simulink model "Add_Frame"  (R2013b)
settings: Solver=FixedStepDiscrete  StartTime=0.0  StopTime=200  RelTol=1e-3
InitFcn:
  | %% DSPBuilder Start
  | alt_dspbuilder_update_model(bdroot)
  | %% DSPBuilder End
StopFcn:
  | ed_out_script
undefined symbols (not defined in the file or in its folder): sigbuilder_block
libraries: allblocks_alteradspbuilder2 x118, simulink x5
(part 2 of 2)

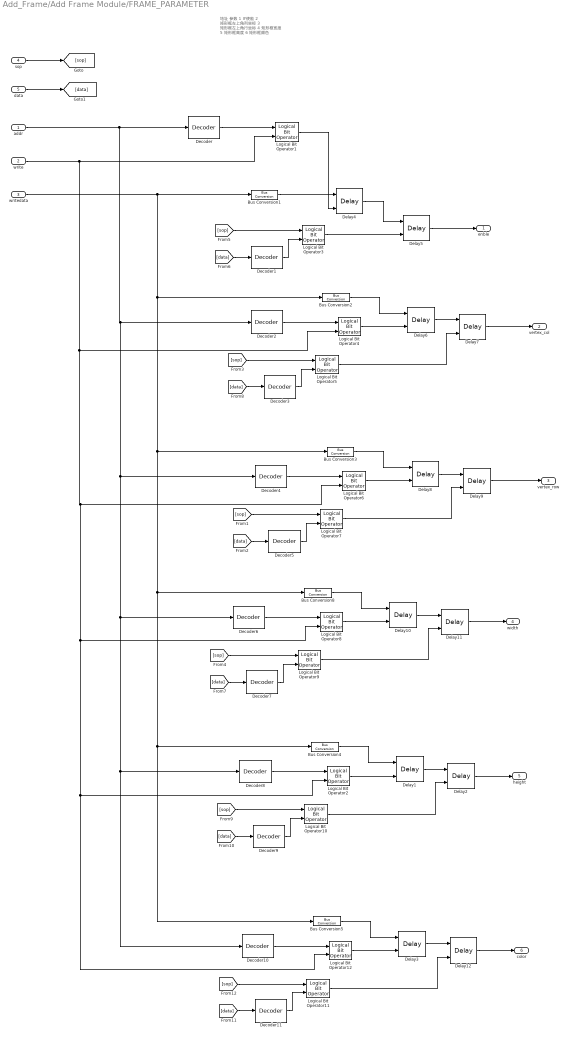
== system Add_Frame/Add Frame Module/FRAME_PARAMETER ==
  note: 地址	参数
      | 1		IP使能
      | 2		矩形框左上角列坐标
      | 3		矩形框左上角行坐标
      | 4		矩形框宽度
      | 5		矩形框高度
      | 6		矩形框颜色
  addr : Inport
  write : Inport  Port=2
  writedata : Inport  Port=3
  sop : Inport  Port=4
  data : Inport  Port=5
  Bus Conversion1 : allblocks_alteradspbuilder2/Bus Conversion  BusType=Unsigned Integer  ibwl=32  ibwr=1  bwl=1  bwr=1  bitToConnectToOutputLSB=0  round=off  saturate=off  pipeline_display=0
  Bus Conversion{2..4,8} (4 alike) : allblocks_alteradspbuilder2/Bus Conversion  BusType=Unsigned Integer  ibwl=32  ibwr=1  bwl=16  bwr=1  bitToConnectToOutputLSB=0  round=off  saturate=off  pipeline_display=0
  Bus Conversion5 : allblocks_alteradspbuilder2/Bus Conversion  BusType=Unsigned Integer  ibwl=32  ibwr=1  bwl=3  bwr=1  bitToConnectToOutputLSB=0  round=off  saturate=off  pipeline_display=0
  Decoder : allblocks_alteradspbuilder2/Decoder  BusType=Unsigned Integer  bwl=3  bwr=2  registered=on  pipeline_display=1  value=1
  Decoder{1,3,5,7,9,11} (6 alike) : allblocks_alteradspbuilder2/Decoder  BusType=Unsigned Integer  bwl=24  bwr=2  registered=off  pipeline_display=0  value=15
  Decoder10 : allblocks_alteradspbuilder2/Decoder  BusType=Unsigned Integer  bwl=3  bwr=2  registered=on  pipeline_display=1  value=6
  Decoder2 : allblocks_alteradspbuilder2/Decoder  BusType=Unsigned Integer  bwl=3  bwr=2  registered=on  pipeline_display=1  value=2
  Decoder4 : allblocks_alteradspbuilder2/Decoder  BusType=Unsigned Integer  bwl=3  bwr=2  registered=on  pipeline_display=1  value=3
  Decoder6 : allblocks_alteradspbuilder2/Decoder  BusType=Unsigned Integer  bwl=3  bwr=2  registered=on  pipeline_display=1  value=4
  Decoder8 : allblocks_alteradspbuilder2/Decoder  BusType=Unsigned Integer  bwl=3  bwr=2  registered=on  pipeline_display=1  value=5
  Delay1 : allblocks_alteradspbuilder2/Delay  pipeline=1  pipeline_display=1  ClockPhase=1  use_ena=on  use_sclr=off  allowFloatingPointOverride=on  logOutputs=off  logFile=E:\FPGA\SOC\Quartus\quartus\dsp_builder\design\VIP_LIB\Add_Frame\tb_Add_Frame\Add%5FFrame_Add+Frame+Module_FRAME%5FPARAMETER_Delay1.fixedpointlog  use_init=on  reset_value=10
  Delay10 : allblocks_alteradspbuilder2/Delay  pipeline=1  pipeline_display=1  ClockPhase=1  use_ena=on  use_sclr=off  allowFloatingPointOverride=on  logOutputs=off  logFile=E:\FPGA\SOC\Quartus\quartus\dsp_builder\design\VIP_LIB\Add_Frame\tb_Add_Frame\Add%5FFrame_Add+Frame+Module_FRAME%5FPARAMETER_Delay10.fixedpointlog  use_init=on  reset_value=10
  Delay11 : allblocks_alteradspbuilder2/Delay  pipeline=1  pipeline_display=1  ClockPhase=1  use_ena=on  use_sclr=off  allowFloatingPointOverride=on  logOutputs=off  logFile=E:\FPGA\SOC\Quartus\quartus\dsp_builder\design\VIP_LIB\Add_Frame\tb_Add_Frame\Add%5FFrame_Add+Frame+Module_FRAME%5FPARAMETER_Delay11.fixedpointlog  use_init=on  reset_value=10
  Delay12 : allblocks_alteradspbuilder2/Delay  pipeline=1  pipeline_display=1  ClockPhase=1  use_ena=on  use_sclr=off  allowFloatingPointOverride=on  logOutputs=off  logFile=E:\FPGA\SOC\Quartus\quartus\dsp_builder\design\VIP_LIB\Add_Frame\tb_Add_Frame\Add%5FFrame_Add+Frame+Module_FRAME%5FPARAMETER_Delay12.fixedpointlog  use_init=on  reset_value=0
  Delay2 : allblocks_alteradspbuilder2/Delay  pipeline=1  pipeline_display=1  ClockPhase=1  use_ena=on  use_sclr=off  allowFloatingPointOverride=on  logOutputs=off  logFile=E:\FPGA\SOC\Quartus\quartus\dsp_builder\design\VIP_LIB\Add_Frame\tb_Add_Frame\Add%5FFrame_Add+Frame+Module_FRAME%5FPARAMETER_Delay2.fixedpointlog  use_init=on  reset_value=10
  Delay3 : allblocks_alteradspbuilder2/Delay  pipeline=1  pipeline_display=1  ClockPhase=1  use_ena=on  use_sclr=off  allowFloatingPointOverride=on  logOutputs=off  logFile=E:\FPGA\SOC\Quartus\quartus\dsp_builder\design\VIP_LIB\Add_Frame\tb_Add_Frame\Add%5FFrame_Add+Frame+Module_FRAME%5FPARAMETER_Delay3.fixedpointlog  use_init=on  reset_value=0
  Delay4 : allblocks_alteradspbuilder2/Delay  pipeline=1  pipeline_display=1  ClockPhase=1  use_ena=on  use_sclr=off  allowFloatingPointOverride=on  logOutputs=off  logFile=E:\FPGA\SOC\Quartus\quartus\dsp_builder\design\VIP_LIB\Add_Frame\tb_Add_Frame\Add%5FFrame_Add+Frame+Module_FRAME%5FPARAMETER_Delay4.fixedpointlog  use_init=on  reset_value=0
  Delay5 : allblocks_alteradspbuilder2/Delay  pipeline=1  pipeline_display=1  ClockPhase=1  use_ena=on  use_sclr=off  allowFloatingPointOverride=on  logOutputs=off  logFile=E:\FPGA\SOC\Quartus\quartus\dsp_builder\design\VIP_LIB\Add_Frame\tb_Add_Frame\Add%5FFrame_Add+Frame+Module_FRAME%5FPARAMETER_Delay5.fixedpointlog  use_init=on  reset_value=0
  Delay6 : allblocks_alteradspbuilder2/Delay  pipeline=1  pipeline_display=1  ClockPhase=1  use_ena=on  use_sclr=off  allowFloatingPointOverride=on  logOutputs=off  logFile=E:\FPGA\SOC\Quartus\quartus\dsp_builder\design\VIP_LIB\Add_Frame\tb_Add_Frame\Add%5FFrame_Add+Frame+Module_FRAME%5FPARAMETER_Delay6.fixedpointlog  use_init=on  reset_value=10
  Delay7 : allblocks_alteradspbuilder2/Delay  pipeline=1  pipeline_display=1  ClockPhase=1  use_ena=on  use_sclr=off  allowFloatingPointOverride=on  logOutputs=off  logFile=E:\FPGA\SOC\Quartus\quartus\dsp_builder\design\VIP_LIB\Add_Frame\tb_Add_Frame\Add%5FFrame_Add+Frame+Module_FRAME%5FPARAMETER_Delay7.fixedpointlog  use_init=on  reset_value=10
  Delay8 : allblocks_alteradspbuilder2/Delay  pipeline=1  pipeline_display=1  ClockPhase=1  use_ena=on  use_sclr=off  allowFloatingPointOverride=on  logOutputs=off  logFile=E:\FPGA\SOC\Quartus\quartus\dsp_builder\design\VIP_LIB\Add_Frame\tb_Add_Frame\Add%5FFrame_Add+Frame+Module_FRAME%5FPARAMETER_Delay8.fixedpointlog  use_init=on  reset_value=10
  Delay9 : allblocks_alteradspbuilder2/Delay  pipeline=1  pipeline_display=1  ClockPhase=1  use_ena=on  use_sclr=off  allowFloatingPointOverride=on  logOutputs=off  logFile=E:\FPGA\SOC\Quartus\quartus\dsp_builder\design\VIP_LIB\Add_Frame\tb_Add_Frame\Add%5FFrame_Add+Frame+Module_FRAME%5FPARAMETER_Delay9.fixedpointlog  use_init=on  reset_value=10
  Logical Bit Operator{1..12} (12 alike) : allblocks_alteradspbuilder2/Logical Bit Operator  LogicalOperator=AND  user_inputs=2  pipeline_display=0
  enble : Outport
  vertex_col : Outport  Port=2
  vertex_row : Outport  Port=3
  width : Outport  Port=4
  height : Outport  Port=5
  color : Outport  Port=6
  wires:
  Decoder/1 -> Logical Bit Operator1/1
  [data] -> Decoder1/1
  [sop] -> Logical Bit Operator3/1
  Decoder1/1 -> Logical Bit Operator3/2
  Logical Bit Operator1/1 -> Delay4/2
  Logical Bit Operator3/1 -> Delay5/2
  Bus Conversion1/1 -> Delay4/1
  Decoder2/1 -> Logical Bit Operator4/1
  Delay6/1 -> Delay7/1
  [data] -> Decoder3/1
  [sop] -> Logical Bit Operator5/1
  Decoder3/1 -> Logical Bit Operator5/2
  Logical Bit Operator4/1 -> Delay6/2
  Bus Conversion2/1 -> Delay6/1
  Decoder4/1 -> Logical Bit Operator6/1
  [data] -> Decoder5/1
  [sop] -> Logical Bit Operator7/1
  Decoder5/1 -> Logical Bit Operator7/2
  Logical Bit Operator7/1 -> Delay9/2
  Logical Bit Operator6/1 -> Delay8/2
  Bus Conversion3/1 -> Delay8/1
  writedata/1 -> Bus Conversion5/1, Bus Conversion4/1, Bus Conversion8/1, Bus Conversion3/1, Bus Conversion2/1, Bus Conversion1/1
  Decoder6/1 -> Logical Bit Operator8/1
  Delay10/1 -> Delay11/1
  [data] -> Decoder7/1
  [sop] -> Logical Bit Operator9/1
  Decoder7/1 -> Logical Bit Operator9/2
  Logical Bit Operator9/1 -> Delay11/2
  Logical Bit Operator8/1 -> Delay10/2
  Bus Conversion8/1 -> Delay10/1
  sop/1 -> [sop]
  data/1 -> [data]
  Delay4/1 -> Delay5/1
  Delay5/1 -> enble/1
  Logical Bit Operator5/1 -> Delay7/2
  Delay7/1 -> vertex_col/1
  Delay8/1 -> Delay9/1
  Delay9/1 -> vertex_row/1
  Delay11/1 -> width/1
  Decoder8/1 -> Logical Bit Operator2/1
  Delay1/1 -> Delay2/1
  [data] -> Decoder9/1
  [sop] -> Logical Bit Operator10/1
  Decoder9/1 -> Logical Bit Operator10/2
  Logical Bit Operator10/1 -> Delay2/2
  Logical Bit Operator2/1 -> Delay1/2
  Bus Conversion4/1 -> Delay1/1
  Delay2/1 -> height/1
  write/1 -> Logical Bit Operator1/2, Logical Bit Operator12/2, Logical Bit Operator2/2, Logical Bit Operator8/2, Logical Bit Operator6/2, Logical Bit Operator4/2
  Decoder10/1 -> Logical Bit Operator12/1
  Delay3/1 -> Delay12/1
  [data] -> Decoder11/1
  [sop] -> Logical Bit Operator11/1
  Decoder11/1 -> Logical Bit Operator11/2
  Logical Bit Operator11/1 -> Delay12/2
  Logical Bit Operator12/1 -> Delay3/2
  Bus Conversion5/1 -> Delay3/1
  Delay12/1 -> color/1
  addr/1 -> Decoder/1, Decoder4/1, Decoder10/1, Decoder8/1, Decoder6/1, Decoder2/1
